simulink model "first"  (R2021b)
settings: Solver=FixedStepDiscrete  StartTime=0.0  StopTime=200  FixedStep=0.01  RelTol=1e-3
libraries: simulink x1
settings Model: Creator=fredric  LastModifiedBy=fredric
settings DataIOCC: InspectSignalLogs=on

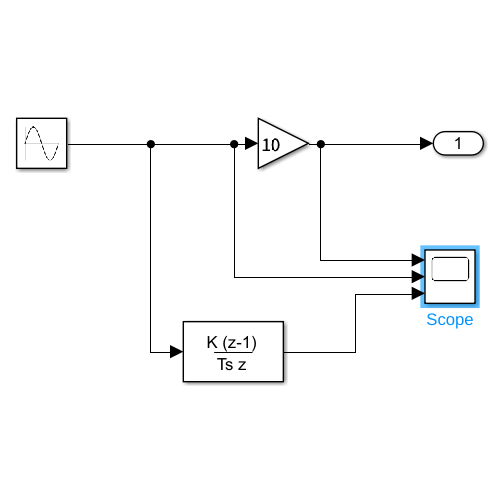
[thumbnail: Simulink's stored preview of the top-level diagram]
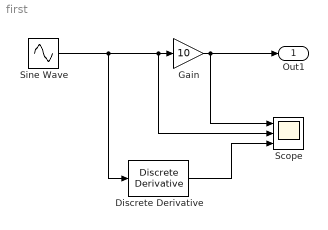
== system first ==
  Discrete Derivative : simulink/Discrete/Discrete Derivative  gainval=1.0  ICPrevScaledInput=0.0  OutMin=[]  OutMax=[]  OutDataType=fixdt(1, 16)  OutScaling=2^-10  DoSatur=off
  Gain : Gain  Gain=10
  Scope : Scope  NumInputPorts=3
  Sine Wave : Sin  SampleTime=0
  Out1 : Outport
  wires:
  Sine Wave/1 -> Discrete Derivative/1, Scope/2, Gain/1
  Gain/1 -> Scope/1, Out1/1
  Discrete Derivative/1 -> Scope/3
